simulink model "AFE_feed_VSI"  (Simulink 8.2)
settings: Solver=ode23tb  StartTime=0  StopTime=1  MaxStep=.5e-6  RelTol=1e-4  AbsTol=1e-5
values from neighbouring files (symbols this model uses):
  Ca = 41.308e-6    (= 4.1308e-05)    [VSI_AFE_parameters_stable.m]    (also in VSI_AFE_parameters_unstable.m)
  Cc = 41.308e-6    (= 4.1308e-05)    [VSI_AFE_parameters_stable.m]    (also in VSI_AFE_parameters_unstable.m)
  Cdc_afe = 35e-6    (= 3.5e-05)    [VSI_AFE_parameters_stable.m]    (also in VSI_AFE_parameters_unstable.m)
  Cdc_vsi = 10e-6    (= 1e-05)    [VSI_AFE_parameters_stable.m]    (also in VSI_AFE_parameters_unstable.m)
  DeadTime = 0.5e-6    (= 5e-07)    [VSI_AFE_parameters_stable.m]    (also in VSI_AFE_parameters_unstable.m)
  f = 400    [VSI_AFE_parameters_stable.m]    (also in VSI_AFE_parameters_unstable.m)
  FWPI_a1 = 26.7622    [VSI_AFE_parameters_stable.m]    (also in VSI_AFE_parameters_unstable.m)
  FWPI_a2 = -24.9784    [VSI_AFE_parameters_stable.m]    (also in VSI_AFE_parameters_unstable.m)
  Kii_AFE = 2.5598*270    (= 691.146)    [VSI_AFE_parameters_stable.m]    (also in VSI_AFE_parameters_unstable.m)
  Kii_VSI = 18.62*270    (= 5027.4)    [VSI_AFE_parameters_stable.m]    (also in VSI_AFE_parameters_unstable.m = 1507.95)
  Kiv_AFE = 6.9813    [VSI_AFE_parameters_stable.m]    (also in VSI_AFE_parameters_unstable.m = 3.49)
  Kiv_VSI = 125.6637    [VSI_AFE_parameters_stable.m]    (also in VSI_AFE_parameters_unstable.m = 41.89)
  Kpi_AFE = 0.0119*270    (= 3.213)    [VSI_AFE_parameters_stable.m]    (also in VSI_AFE_parameters_unstable.m)
  Kpi_VSI = 0.0102*270    (= 2.754)    [VSI_AFE_parameters_stable.m]    (also in VSI_AFE_parameters_unstable.m)
  Kpv_AFE = 0.022    [VSI_AFE_parameters_stable.m]    (also in VSI_AFE_parameters_unstable.m = 0.011)
  Kpv_VSI = 0.0779    [VSI_AFE_parameters_stable.m]    (also in VSI_AFE_parameters_unstable.m = 0.026)
  La = 962e-6    (= 0.000962)    [VSI_AFE_parameters_stable.m]    (also in VSI_AFE_parameters_unstable.m)
  Lb = 985e-6    (= 0.000985)    [VSI_AFE_parameters_stable.m]    (also in VSI_AFE_parameters_unstable.m)
  Lboost_a = 474e-6    (= 0.000474)    [VSI_AFE_parameters_stable.m]    (also in VSI_AFE_parameters_unstable.m)
  Lboost_b = 471e-6    (= 0.000471)    [VSI_AFE_parameters_stable.m]    (also in VSI_AFE_parameters_unstable.m)
  Lboost_c = 463e-6    (= 0.000463)    [VSI_AFE_parameters_stable.m]    (also in VSI_AFE_parameters_unstable.m)
  Lc = 972e-6    (= 0.000972)    [VSI_AFE_parameters_stable.m]    (also in VSI_AFE_parameters_unstable.m)
  LCa = 0.61e-6    (= 6.1e-07)    [VSI_AFE_parameters_stable.m]    (also in VSI_AFE_parameters_unstable.m)
  LCb = 0.61e-6    (= 6.1e-07)    [VSI_AFE_parameters_stable.m]    (also in VSI_AFE_parameters_unstable.m)
  LCc = 0.63e-6    (= 6.3e-07)    [VSI_AFE_parameters_stable.m]    (also in VSI_AFE_parameters_unstable.m)
  PWM_Cycle = 4000    [VSI_AFE_parameters_stable.m]    (also in VSI_AFE_parameters_unstable.m)
  R = 10    [VSI_AFE_parameters_stable.m]    (also in VSI_AFE_parameters_unstable.m)
  RCa = 0.051    [VSI_AFE_parameters_stable.m]    (also in VSI_AFE_parameters_unstable.m)
  RCb = 0.054    [VSI_AFE_parameters_stable.m]    (also in VSI_AFE_parameters_unstable.m)
  RCc = 0.052    [VSI_AFE_parameters_stable.m]    (also in VSI_AFE_parameters_unstable.m)
  RCdc_afe = 0.049    [VSI_AFE_parameters_stable.m]    (also in VSI_AFE_parameters_unstable.m)
  RCdc_vsi = 0.046    [VSI_AFE_parameters_stable.m]    (also in VSI_AFE_parameters_unstable.m)
  RLa = 0.123    [VSI_AFE_parameters_stable.m]    (also in VSI_AFE_parameters_unstable.m)
  RLb = 0.132    [VSI_AFE_parameters_stable.m]    (also in VSI_AFE_parameters_unstable.m)
  RLboost_a = 0.080    (= 0.08)    [VSI_AFE_parameters_stable.m]    (also in VSI_AFE_parameters_unstable.m)
  RLboost_c = 0.110    (= 0.11)    [VSI_AFE_parameters_stable.m]    (also in VSI_AFE_parameters_unstable.m)
  RLc = 0.089    [VSI_AFE_parameters_stable.m]    (also in VSI_AFE_parameters_unstable.m)
  Vfd = 0.75    [VSI_AFE_parameters_stable.m]    (also in VSI_AFE_parameters_unstable.m)
  Vfs = 1.0    (= 1)    [VSI_AFE_parameters_stable.m]    (also in VSI_AFE_parameters_unstable.m)
  Vsm = Vse*sqrt(2)    [VSI_AFE_parameters_stable.m]    (also in VSI_AFE_parameters_unstable.m)
undefined symbols (not defined in the file or in its folder): Cdc, Ldc
libraries: powerlib x42, cstblocks x10, simulink x4, powerlib_extras x1
settings Model: Creator=marko  LastModifiedBy=wenbo
settings SolverCC: MaxConsecutiveMinStep=10  ZeroCrossAlgorithm=Adaptive  AlgebraicLoopSolver=LineSearch
settings DataIOCC: LimitDataPoints=off  SaveOutput=off  SignalLogging=off  DSMLogging=off  SaveTime=off
settings DebuggingCC: IgnoredZcDiagnostic=none  FcnCallInpInsideContextMsg=EnableAllAsWarning

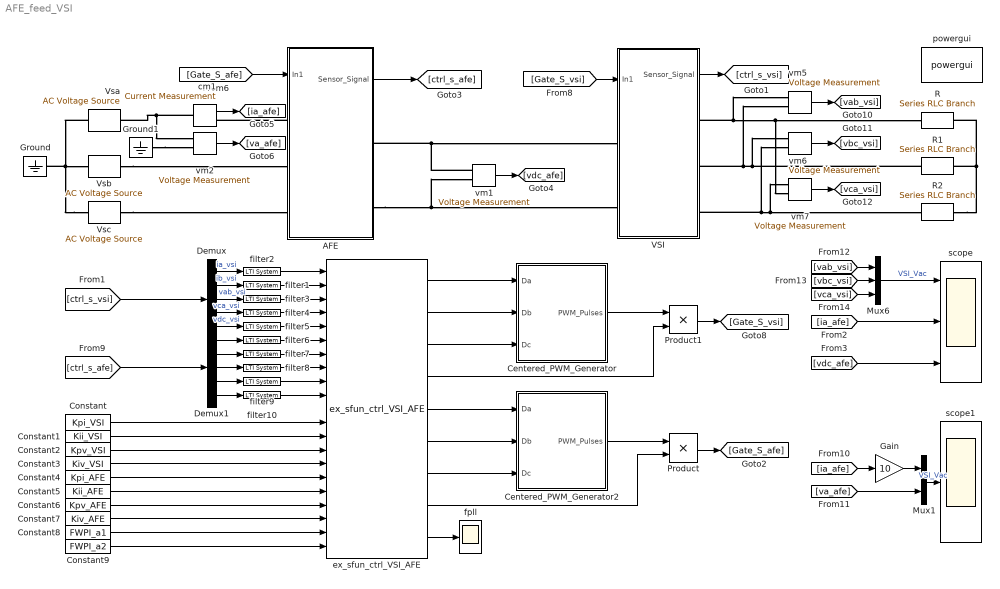
== system AFE_feed_VSI ==
  AFE : Subsystem
  Centered_PWM_Generator : Subsystem
  Centered_PWM_Generator2 : Subsystem
  Constant : Constant  Value=Kpi_VSI
  Constant1 : Constant  Value=Kii_VSI
  Constant2 : Constant  Value=Kpv_VSI
  Constant3 : Constant  Value=Kiv_VSI
  Constant4 : Constant  Value=Kpi_AFE
  Constant5 : Constant  Value=Kii_AFE
  Constant6 : Constant  Value=Kpv_AFE
  Constant7 : Constant  Value=Kiv_AFE
  Constant8 : Constant  Value=FWPI_a1
  Constant9 : Constant  Value=FWPI_a2
  Demux : Demux  Outputs=5
  Demux1 : Demux  Outputs=5
  Gain : Gain  Gain=10
  Ground : powerlib/Elements/Ground  LConnTagsString=a
  Ground1 : powerlib/Elements/Ground  LConnTagsString=a
  Mux1 : Mux  Inputs=2
  Mux6 : Mux  Inputs=3
  Product : Product  RndMeth=Zero
  Product1 : Product  RndMeth=Zero
  R : powerlib/Elements/Series RLC Branch  LConnTagsString=__new0  RConnTagsString=__new0  BranchType=R  Resistance=R  Inductance=Ldc  SetiL0=off  InitialCurrent=0  Capacitance=Cdc  Setx0=off  InitialVoltage=0  Measurements=None
  R1 : powerlib/Elements/Series RLC Branch  LConnTagsString=__new0  RConnTagsString=__new0  BranchType=R  Resistance=R  Inductance=Ldc  SetiL0=off  InitialCurrent=0  Capacitance=Cdc  Setx0=off  InitialVoltage=0  Measurements=None
  R2 : powerlib/Elements/Series RLC Branch  LConnTagsString=__new0  RConnTagsString=__new0  BranchType=R  Resistance=R  Inductance=Ldc  SetiL0=off  InitialCurrent=0  Capacitance=Cdc  Setx0=off  InitialVoltage=0  Measurements=None
  VSI : Subsystem
  Vsa : powerlib/Electrical Sources/AC Voltage Source  Amplitude=Vsm  Phase=90  Frequency=f  SampleTime=0  Measurements=None
  Vsb : powerlib/Electrical Sources/AC Voltage Source  Amplitude=Vsm  Phase=90-120  Frequency=f  SampleTime=0  Measurements=None
  Vsc : powerlib/Electrical Sources/AC Voltage Source  Amplitude=Vsm  Phase=90+120  Frequency=f  SampleTime=0  Measurements=None
  cm1 : powerlib/Measurements/Current Measurement  PhasorSimulation=off  OutputType=Complex  PSBequivalent=0
  ex_sfun_ctrl_VSI_AFE : S-Function  FunctionName=ex_sfun_ctrl_VSI_AFE  EnableBusSupport=off
  filter{1..3,6..8} (6 alike) : cstblocks/LTI System  sys=tf_i_filter  IC=[]
  filter{4..5,9..10} (4 alike) : cstblocks/LTI System  sys=tf_v_filter  IC=[]
  fpll : Scope
      settings: YMin=-500  YMax=50  SaveName=ia_L1
  powergui : powerlib/powergui  Priority=1  SimulationMode=Continuous  SolverType=Tustin  SampleTime=50e-6  frequency=60  SPID=on  DisableSnubberDevices=off  DisableRonSwitches=off  DisableVfSwitches=off  SwTol=0  Interpol=off  DisplayEquations=off  frequencyindice=0  Pbase=100e6  ErrMax=1e-4  Iterations=50  UnitsV=kV  UnitsW=MW  FunctionMessages=off  echomessages=off  HookPort=off  EnableUseOfTLC=off  x0status=blocks  RestoreLinks=warning  ResistiveCurrentMeasurement=off  Frange=[0:2:500]  Ylog=off  Xlog=on  ShowGrid=off  save=off  variable=ZData  structure=ia_L  ZoomFFT=on  StartTime=0.1  cycles=1  DisplayStyle=1  fundamental=400  FreqAxis=off  MaxFrequency=100000  frequencyindicesteady=400  RmsSteady=1  display=off  Ts=0  methode=off
  scope : Scope  NumInputPorts=3
      settings: YMin=-200~-15~0  YMax=200~30~450  SaveName=va_ia  MaxDataPoints=2000000
  scope1 : Scope
      settings: YMin=-800  YMax=900  SaveName=va_ia1  MaxDataPoints=2000000
  vm{1..2,5..7} (5 alike) : powerlib/Measurements/Voltage Measurement  PhasorSimulation=off  OutputType=Complex  PSBequivalent=0
  wires:
  vm5/1 -> [vab_vsi]
  vm6/1 -> [vbc_vsi]
  vm7/1 -> [vca_vsi]
  [vab_vsi] -> Mux6/1
  [vbc_vsi] -> Mux6/2
  [vca_vsi] -> Mux6/3
  Mux6/1 -> scope/1  "VSI_Vac"
  VSI/1(Sensor_Signal) -> [ctrl_s_vsi]
  [Gate_S_vsi] -> VSI/1(In1)
  [ctrl_s_afe] -> Demux1/1
  [Gate_S_afe] -> AFE/1(In1)
  AFE/1(Sensor_Signal) -> [ctrl_s_afe]
  ex_sfun_ctrl_VSI_AFE/1 -> Centered_PWM_Generator/1(Da)
  ex_sfun_ctrl_VSI_AFE/2 -> Centered_PWM_Generator/2(Db)
  ex_sfun_ctrl_VSI_AFE/3 -> Centered_PWM_Generator/3(Dc)
  Centered_PWM_Generator2/1(PWM_Pulses) -> Product/1
  Product/1 -> [Gate_S_afe]
  vm1/1 -> [vdc_afe]
  cm1/1 -> [ia_afe]
  [ia_afe] -> scope/2
  [vdc_afe] -> scope/3
  [ctrl_s_vsi] -> Demux/1
  Demux/1 -> filter2/1  "ia_vsi"
  Demux/2 -> filter1/1  "ib_vsi"
  Demux/3 -> filter3/1  "vab_vsi"
  Demux/4 -> filter4/1  "vca_vsi"
  Demux/5 -> filter5/1  "vdc_vsi"
  Demux1/1 -> filter6/1
  Demux1/2 -> filter7/1
  Demux1/3 -> filter8/1
  Demux1/4 -> filter9/1
  Demux1/5 -> filter10/1
  Constant/1 -> ex_sfun_ctrl_VSI_AFE/12
  Constant1/1 -> ex_sfun_ctrl_VSI_AFE/13
  Constant2/1 -> ex_sfun_ctrl_VSI_AFE/14
  Constant3/1 -> ex_sfun_ctrl_VSI_AFE/15
  Constant4/1 -> ex_sfun_ctrl_VSI_AFE/16
  Constant5/1 -> ex_sfun_ctrl_VSI_AFE/17
  Constant6/1 -> ex_sfun_ctrl_VSI_AFE/18
  Constant7/1 -> ex_sfun_ctrl_VSI_AFE/19
  Constant8/1 -> ex_sfun_ctrl_VSI_AFE/20
  Constant9/1 -> ex_sfun_ctrl_VSI_AFE/21
  filter2/1 -> ex_sfun_ctrl_VSI_AFE/1
  filter1/1 -> ex_sfun_ctrl_VSI_AFE/2
  filter3/1 -> ex_sfun_ctrl_VSI_AFE/3
  filter4/1 -> ex_sfun_ctrl_VSI_AFE/4
  filter5/1 -> ex_sfun_ctrl_VSI_AFE/5
  filter6/1 -> ex_sfun_ctrl_VSI_AFE/6
  filter7/1 -> ex_sfun_ctrl_VSI_AFE/7
  filter8/1 -> ex_sfun_ctrl_VSI_AFE/8
  filter9/1 -> ex_sfun_ctrl_VSI_AFE/9
  filter10/1 -> ex_sfun_ctrl_VSI_AFE/10
  vm2/1 -> [va_afe]
  ex_sfun_ctrl_VSI_AFE/9 -> fpll/1
  ex_sfun_ctrl_VSI_AFE/5 -> Centered_PWM_Generator2/1(Da)
  ex_sfun_ctrl_VSI_AFE/6 -> Centered_PWM_Generator2/2(Db)
  ex_sfun_ctrl_VSI_AFE/7 -> Centered_PWM_Generator2/3(Dc)
  ex_sfun_ctrl_VSI_AFE/8 -> Product/2
  Product1/1 -> [Gate_S_vsi]
  Centered_PWM_Generator/1(PWM_Pulses) -> Product1/1
  ex_sfun_ctrl_VSI_AFE/4 -> Product1/2
  Mux1/1 -> scope1/1  "VSI_Vac"
  [ia_afe] -> Gain/1
  [va_afe] -> Mux1/2
  Gain/1 -> Mux1/1
  connections:
  VSI/RConn1 -- vm5/LConn1 -- R/RConn1 -- vm7/LConn2
  R1/RConn1 -- VSI/RConn2 -- vm5/LConn2 -- vm6/LConn1
  VSI/RConn3 -- vm6/LConn2 -- R2/RConn1 -- vm7/LConn1
  AFE/RConn2 -- VSI/LConn2 -- vm1/LConn2
  Vsc/LConn1 -- Vsb/LConn1 -- Vsa/LConn1 -- Ground/LConn1
  Vsb/RConn1 -- AFE/LConn2
  Vsc/RConn1 -- AFE/LConn3
  AFE/LConn1 -- cm1/RConn1
  cm1/LConn1 -- Vsa/RConn1 -- vm2/LConn1
  Ground1/LConn1 -- vm2/LConn2
  R2/LConn1 -- R/LConn1 -- R1/LConn1
  vm1/LConn1 -- VSI/LConn1 -- AFE/RConn1

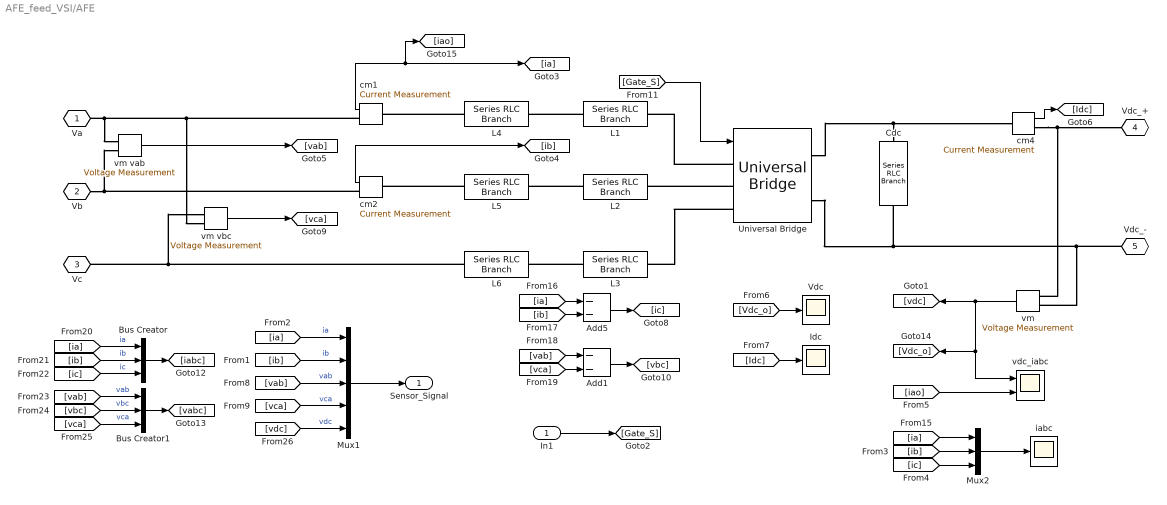
== system AFE_feed_VSI/AFE ==
  In1 : Inport
  Add1 : Sum  Inputs=--
  Add5 : Sum  Inputs=--
  Bus Creator : BusCreator  Inputs=3
  Bus Creator1 : BusCreator  Inputs=3
  Cdc : powerlib/Elements/Series RLC Branch  LConnTagsString=__new0  RConnTagsString=__new0  BranchType=RC  Resistance=RCdc_afe  Inductance=Ldc  SetiL0=off  InitialCurrent=0  Capacitance=Cdc_afe  Setx0=off  InitialVoltage=0  Measurements=None
  Idc : Scope
      settings: YMin=1.813  YMax=1.8195  SaveName=vdc_matlab1
  L1 : powerlib/Elements/Series RLC Branch  LConnTagsString=__new0  RConnTagsString=__new0  BranchType=L  Resistance=RLa  Inductance=Lboost_a  SetiL0=off  InitialCurrent=0  Capacitance=1e-6  Setx0=off  InitialVoltage=0  Measurements=None
  L2 : powerlib/Elements/Series RLC Branch  LConnTagsString=__new0  RConnTagsString=__new0  BranchType=L  Resistance=RLa  Inductance=Lboost_b  SetiL0=off  InitialCurrent=0  Capacitance=1e-6  Setx0=off  InitialVoltage=0  Measurements=None
  L3 : powerlib/Elements/Series RLC Branch  LConnTagsString=__new0  RConnTagsString=__new0  BranchType=L  Resistance=RLa  Inductance=Lboost_c  SetiL0=off  InitialCurrent=0  Capacitance=1e-6  Setx0=off  InitialVoltage=0  Measurements=None
  L4 : powerlib/Elements/Series RLC Branch  LConnTagsString=__new0  RConnTagsString=__new0  BranchType=R  Resistance=RLboost_a  Inductance=La  SetiL0=off  InitialCurrent=0  Capacitance=1e-6  Setx0=off  InitialVoltage=0  Measurements=None
  L5 : powerlib/Elements/Series RLC Branch  LConnTagsString=__new0  RConnTagsString=__new0  BranchType=R  Resistance=Lboost_b  Inductance=La  SetiL0=off  InitialCurrent=0  Capacitance=1e-6  Setx0=off  InitialVoltage=0  Measurements=None
  L6 : powerlib/Elements/Series RLC Branch  LConnTagsString=__new0  RConnTagsString=__new0  BranchType=R  Resistance=RLboost_c  Inductance=La  SetiL0=off  InitialCurrent=0  Capacitance=1e-6  Setx0=off  InitialVoltage=0  Measurements=None
  Mux1 : Mux  Inputs=5
  Mux2 : Mux  Inputs=3
  Universal Bridge : powerlib/Power Electronics/Universal Bridge  Arms=3  SnubberResistance=inf  SnubberCapacitance=inf  Device=IGBT / Diodes  Ron=Rsd  Lon=0  ForwardVoltages=[Vfs Vfd]  ForwardVoltage=0  GTOparameters=[ 10e-6 , 20e-6 ]  IGBTparameters=[ 0, 0 ]  Measurements=None  Measurements_2=None  converterType=Rectifier
  Vdc : Scope
      settings: TimeRange=0.3  YMin=0  YMax=300  SaveName=vdc_matlab
  cm1 : powerlib/Measurements/Current Measurement  PhasorSimulation=off  OutputType=Complex  PSBequivalent=0
  cm2 : powerlib/Measurements/Current Measurement  PhasorSimulation=off  OutputType=Complex  PSBequivalent=0
  cm4 : powerlib/Measurements/Current Measurement  PhasorSimulation=off  OutputType=Complex  PSBequivalent=0
  iabc : Scope
      settings: TimeRange=0.06  YMin=-8  YMax=8  SaveName=iabc_L
  vdc_iabc : Scope  NumInputPorts=2
      settings: TimeRange=0.3  YMin=131~-2  YMax=137~2  SaveName=iabc_L1
  vm : powerlib/Measurements/Voltage Measurement  PhasorSimulation=off  OutputType=Complex  PSBequivalent=0
  vm vab : powerlib/Measurements/Voltage Measurement  PhasorSimulation=off  OutputType=Complex  PSBequivalent=0
  vm vbc : powerlib/Measurements/Voltage Measurement  PhasorSimulation=off  OutputType=Complex  PSBequivalent=0
  Va : PMIOPort  Tag=PMCPort  Port=1  Side=Left
  Vb : PMIOPort  Tag=PMCPort  Port=2  Side=Left
  Vc : PMIOPort  Tag=PMCPort  Port=3  Side=Left
  Vdc_+ : PMIOPort  Tag=PMCPort  Port=4  Side=Right
  Vdc_- : PMIOPort  Tag=PMCPort  Port=5  Side=Right
  Sensor_Signal : Outport
  wires:
  [Vdc_o] -> Vdc/1
  [Idc] -> Idc/1
  [Gate_S] -> Universal Bridge/1
  [ia] -> Bus Creator/1  "ia"
  [ib] -> Bus Creator/2  "ib"
  [ic] -> Bus Creator/3  "ic"
  Bus Creator/1 -> [iabc]
  [vab] -> Bus Creator1/1  "vab"
  [vbc] -> Bus Creator1/2  "vbc"
  [vca] -> Bus Creator1/3  "vca"
  Bus Creator1/1 -> [vabc]
  cm4/1 -> [Idc]
  Mux2/1 -> iabc/1
  [ia] -> Mux2/1
  [ib] -> Mux2/2
  [ic] -> Mux2/3
  cm1/1 -> [iao], [ia]
  cm2/1 -> [ib]
  vm vab/1 -> [vab]
  vm vbc/1 -> [vca]
  [iao] -> vdc_iabc/2
  vm/1 -> [Vdc_o], vdc_iabc/1, [vdc]
  [ia] -> Mux1/1  "ia"
  [ib] -> Mux1/2  "ib"
  [vab] -> Mux1/3  "vab"
  [vca] -> Mux1/4  "vca"
  [vdc] -> Mux1/5  "vdc"
  Mux1/1 -> Sensor_Signal/1
  In1/1 -> [Gate_S]
  Add5/1 -> [ic]
  [ia] -> Add5/1
  [ib] -> Add5/2
  Add1/1 -> [vbc]
  [vab] -> Add1/1
  [vca] -> Add1/2
  connections:
  Universal Bridge/LConn1 -- L1/RConn1
  Universal Bridge/LConn2 -- L2/RConn1
  Universal Bridge/LConn3 -- L3/RConn1
  vm vab/LConn1 -- cm1/RConn1 -- vm vbc/LConn2 -- Va/RConn1
  cm2/RConn1 -- Vb/RConn1 -- vm vab/LConn2
  L6/LConn1 -- Vc/RConn1 -- vm vbc/LConn1
  cm4/RConn1 -- Vdc_+/RConn1 -- vm/LConn1
  Vdc_-/RConn1 -- Universal Bridge/RConn2 -- Cdc/RConn1 -- vm/LConn2
  L1/LConn1 -- L4/RConn1
  L4/LConn1 -- cm1/LConn1
  L2/LConn1 -- L5/RConn1
  L5/LConn1 -- cm2/LConn1
  L3/LConn1 -- L6/RConn1
  Universal Bridge/RConn1 -- cm4/LConn1 -- Cdc/LConn1

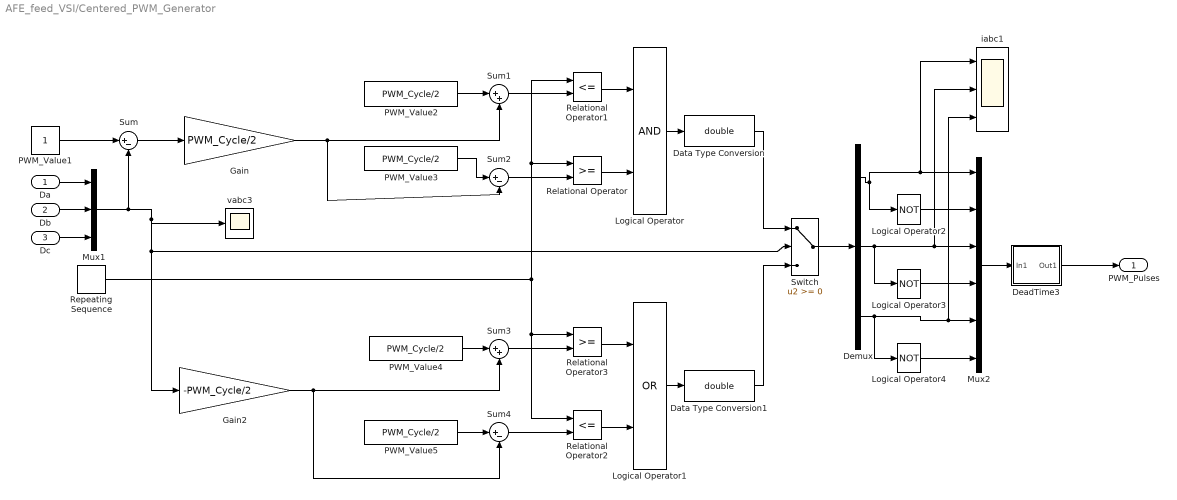
== system AFE_feed_VSI/Centered_PWM_Generator ==
  Da : Inport
  Db : Inport  Port=2
  Dc : Inport  Port=3
  Data Type Conversion : DataTypeConversion  OutDataTypeStr=double
  Data Type Conversion1 : DataTypeConversion  OutDataTypeStr=double
  DeadTime3 : Subsystem
  Demux : Demux  Outputs=3
  Gain : Gain  Gain=PWM_Cycle/2
  Gain2 : Gain  Gain=-PWM_Cycle/2
  Logical Operator : Logic  AllPortsSameDT=off  OutDataTypeStr=boolean
  Logical Operator1 : Logic  Operator=OR  AllPortsSameDT=off  OutDataTypeStr=boolean
  Logical Operator2 : Logic  Operator=NOT  OutDataTypeStr=float('double')
  Logical Operator3 : Logic  Operator=NOT  OutDataTypeStr=float('double')
  Logical Operator4 : Logic  Operator=NOT  OutDataTypeStr=float('double')
  Mux1 : Mux  Inputs=3
  Mux2 : Mux  Inputs=6
  PWM_Value1 : Constant
  PWM_Value{2..5} (4 alike) : Constant  Value=PWM_Cycle/2
  Relational Operator : RelationalOperator  OutDataTypeStr=boolean
  Relational Operator1 : RelationalOperator  Operator=<=  OutDataTypeStr=boolean
  Relational Operator2 : RelationalOperator  Operator=<=  OutDataTypeStr=boolean
  Relational Operator3 : RelationalOperator  OutDataTypeStr=boolean
  Repeating Sequence : simulink/Sources/Repeating Sequence  rep_seq_t="[0  (PWM_Cycle*12.5e-9)]"  rep_seq_y=[0 PWM_Cycle]
  Sum : Sum  Inputs=|+-
  Sum1 : Sum  Inputs=|++
  Sum2 : Sum  Inputs=|+-
  Sum3 : Sum  Inputs=|++
  Sum4 : Sum  Inputs=|+-
  Switch : Switch
  iabc1 : Scope  NumInputPorts=3
      settings: TimeRange=0.02  YMin=-9~-5~-5  YMax=8~5~5  SaveName=iabc_L2
  vabc3 : Scope
      settings: TimeRange=0.01  YMin=0.275  YMax=0.725  SaveName=vabcll1
  PWM_Pulses : Outport
  wires:
  Logical Operator4/1 -> Mux2/6
  Demux/3 -> Logical Operator4/1, Mux2/5, iabc1/3
  Logical Operator3/1 -> Mux2/4
  Demux/2 -> Logical Operator3/1, Mux2/3, iabc1/2
  Logical Operator2/1 -> Mux2/2
  Demux/1 -> Logical Operator2/1, Mux2/1, iabc1/1
  Mux2/1 -> DeadTime3/1(In1)
  Dc/1 -> Mux1/3
  Db/1 -> Mux1/2
  Da/1 -> Mux1/1
  Mux1/1 -> Sum/2, Switch/2, Gain2/1, vabc3/1
  Switch/1 -> Demux/1
  Data Type Conversion1/1 -> Switch/3
  Gain2/1 -> Sum3/2, Sum4/2
  Logical Operator1/1 -> Data Type Conversion1/1
  Relational Operator2/1 -> Logical Operator1/2
  Relational Operator3/1 -> Logical Operator1/1
  Sum3/1 -> Relational Operator3/2
  Sum4/1 -> Relational Operator2/2
  PWM_Value5/1 -> Sum4/1
  PWM_Value4/1 -> Sum3/1
  Data Type Conversion/1 -> Switch/1
  Logical Operator/1 -> Data Type Conversion/1
  Relational Operator/1 -> Logical Operator/2
  Relational Operator1/1 -> Logical Operator/1
  Sum1/1 -> Relational Operator1/2
  Sum2/1 -> Relational Operator/2
  PWM_Value3/1 -> Sum2/1
  Gain/1 -> Sum2/2, Sum1/2
  Sum/1 -> Gain/1
  PWM_Value1/1 -> Sum/1
  Repeating Sequence/1 -> Relational Operator1/1, Relational Operator/1, Relational Operator3/1, Relational Operator2/1
  DeadTime3/1(Out1) -> PWM_Pulses/1
  PWM_Value2/1 -> Sum1/1

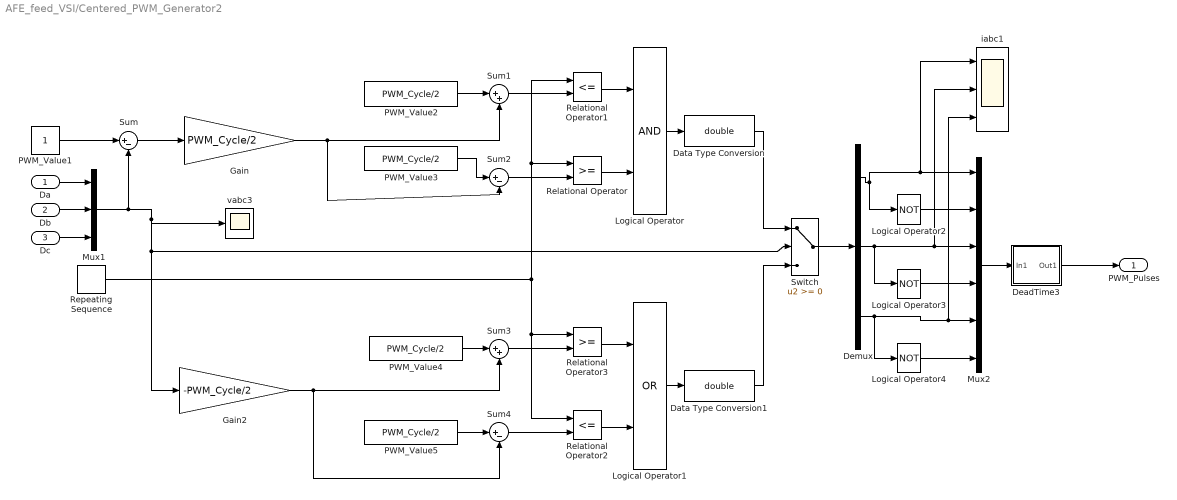
== system AFE_feed_VSI/Centered_PWM_Generator2 ==
  Da : Inport
  Db : Inport  Port=2
  Dc : Inport  Port=3
  Data Type Conversion : DataTypeConversion  OutDataTypeStr=double
  Data Type Conversion1 : DataTypeConversion  OutDataTypeStr=double
  DeadTime3 : Subsystem
  Demux : Demux  Outputs=3
  Gain : Gain  Gain=PWM_Cycle/2
  Gain2 : Gain  Gain=-PWM_Cycle/2
  Logical Operator : Logic  AllPortsSameDT=off  OutDataTypeStr=boolean
  Logical Operator1 : Logic  Operator=OR  AllPortsSameDT=off  OutDataTypeStr=boolean
  Logical Operator2 : Logic  Operator=NOT  OutDataTypeStr=float('double')
  Logical Operator3 : Logic  Operator=NOT  OutDataTypeStr=float('double')
  Logical Operator4 : Logic  Operator=NOT  OutDataTypeStr=float('double')
  Mux1 : Mux  Inputs=3
  Mux2 : Mux  Inputs=6
  PWM_Value1 : Constant
  PWM_Value{2..5} (4 alike) : Constant  Value=PWM_Cycle/2
  Relational Operator : RelationalOperator  OutDataTypeStr=boolean
  Relational Operator1 : RelationalOperator  Operator=<=  OutDataTypeStr=boolean
  Relational Operator2 : RelationalOperator  Operator=<=  OutDataTypeStr=boolean
  Relational Operator3 : RelationalOperator  OutDataTypeStr=boolean
  Repeating Sequence : simulink/Sources/Repeating Sequence  rep_seq_t="[0  (PWM_Cycle*12.5e-9)]"  rep_seq_y=[0 PWM_Cycle]
  Sum : Sum  Inputs=|+-
  Sum1 : Sum  Inputs=|++
  Sum2 : Sum  Inputs=|+-
  Sum3 : Sum  Inputs=|++
  Sum4 : Sum  Inputs=|+-
  Switch : Switch
  iabc1 : Scope  NumInputPorts=3
      settings: TimeRange=0.02  YMin=-9~-5~-5  YMax=8~5~5  SaveName=iabc_L2
  vabc3 : Scope
      settings: TimeRange=0.01  YMin=-35  YMax=35  SaveName=vabcll1
  PWM_Pulses : Outport
  wires:
  Logical Operator4/1 -> Mux2/6
  Demux/3 -> Logical Operator4/1, Mux2/5, iabc1/3
  Logical Operator3/1 -> Mux2/4
  Demux/2 -> Logical Operator3/1, Mux2/3, iabc1/2
  Logical Operator2/1 -> Mux2/2
  Demux/1 -> Logical Operator2/1, Mux2/1, iabc1/1
  Mux2/1 -> DeadTime3/1(In1)
  Dc/1 -> Mux1/3
  Db/1 -> Mux1/2
  Da/1 -> Mux1/1
  Mux1/1 -> Sum/2, Switch/2, Gain2/1, vabc3/1
  Switch/1 -> Demux/1
  Data Type Conversion1/1 -> Switch/3
  Gain2/1 -> Sum3/2, Sum4/2
  Logical Operator1/1 -> Data Type Conversion1/1
  Relational Operator2/1 -> Logical Operator1/2
  Relational Operator3/1 -> Logical Operator1/1
  Sum3/1 -> Relational Operator3/2
  Sum4/1 -> Relational Operator2/2
  PWM_Value5/1 -> Sum4/1
  PWM_Value4/1 -> Sum3/1
  Data Type Conversion/1 -> Switch/1
  Logical Operator/1 -> Data Type Conversion/1
  Relational Operator/1 -> Logical Operator/2
  Relational Operator1/1 -> Logical Operator/1
  Sum1/1 -> Relational Operator1/2
  Sum2/1 -> Relational Operator/2
  PWM_Value3/1 -> Sum2/1
  Gain/1 -> Sum2/2, Sum1/2
  Sum/1 -> Gain/1
  PWM_Value1/1 -> Sum/1
  Repeating Sequence/1 -> Relational Operator1/1, Relational Operator/1, Relational Operator3/1, Relational Operator2/1
  DeadTime3/1(Out1) -> PWM_Pulses/1
  PWM_Value2/1 -> Sum1/1

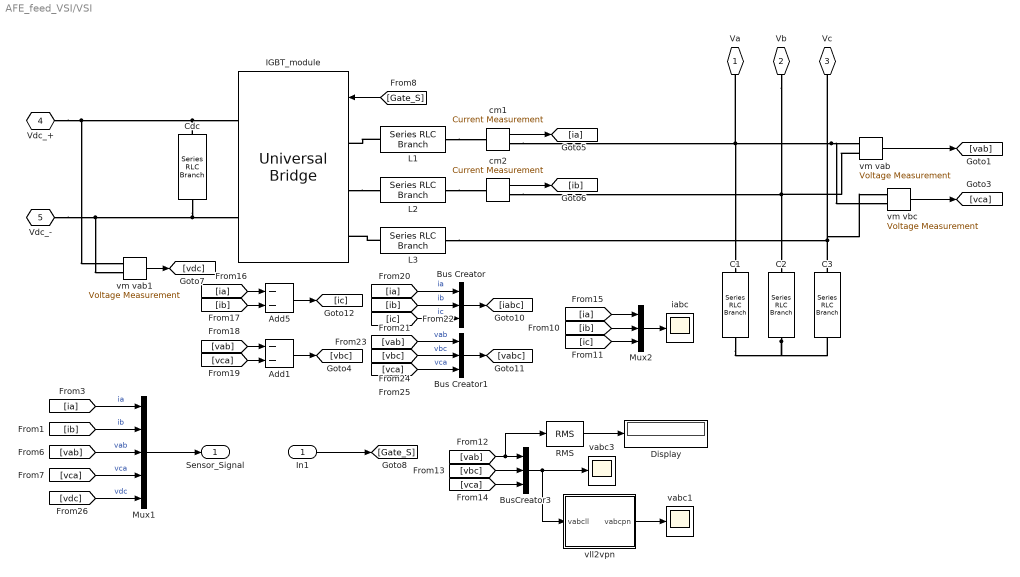
== system AFE_feed_VSI/VSI ==
  In1 : Inport
  Add1 : Sum  Inputs=--
  Add5 : Sum  Inputs=--
  Bus Creator : BusCreator  Inputs=3
  Bus Creator1 : BusCreator  Inputs=3
  BusCreator3 : BusCreator  Inputs=3
  C1 : powerlib/Elements/Series RLC Branch  LConnTagsString=__new0  RConnTagsString=__new0  BranchType=RC  Resistance=RCa  Inductance=LCa  SetiL0=off  InitialCurrent=0  Capacitance=Ca  Setx0=off  InitialVoltage=0  Measurements=None
  C2 : powerlib/Elements/Series RLC Branch  LConnTagsString=__new0  RConnTagsString=__new0  BranchType=RC  Resistance=RCb  Inductance=LCb  SetiL0=off  InitialCurrent=0  Capacitance=Cc  Setx0=off  InitialVoltage=0  Measurements=None
  C3 : powerlib/Elements/Series RLC Branch  LConnTagsString=__new0  RConnTagsString=__new0  BranchType=RC  Resistance=RCc  Inductance=LCc  SetiL0=off  InitialCurrent=0  Capacitance=Cc  Setx0=off  InitialVoltage=0  Measurements=None
  Cdc : powerlib/Elements/Series RLC Branch  LConnTagsString=__new0  RConnTagsString=__new0  BranchType=RC  Resistance=RCdc_vsi  Inductance=Ldc  SetiL0=off  InitialCurrent=0  Capacitance=Cdc_vsi  Setx0=off  InitialVoltage=0  Measurements=None
  Display : Display
  IGBT_module : powerlib/Power Electronics/Universal Bridge  Arms=3  SnubberResistance=inf  SnubberCapacitance=inf  Device=IGBT / Diodes  Ron=Rsd  Lon=0  ForwardVoltages=[Vfs Vfd]  ForwardVoltage=0  GTOparameters=[ 10e-6 , 20e-6 ]  IGBTparameters=[ 0, 0 ]  Measurements=None  Measurements_2=None  converterType=Rectifier
  L1 : powerlib/Elements/Series RLC Branch  LConnTagsString=__new0  RConnTagsString=__new0  BranchType=RL  Resistance=RLa  Inductance=La  SetiL0=off  InitialCurrent=0  Capacitance=1e-6  Setx0=off  InitialVoltage=0  Measurements=None
  L2 : powerlib/Elements/Series RLC Branch  LConnTagsString=__new0  RConnTagsString=__new0  BranchType=RL  Resistance=RLb  Inductance=Lb  SetiL0=off  InitialCurrent=0  Capacitance=1e-6  Setx0=off  InitialVoltage=0  Measurements=None
  L3 : powerlib/Elements/Series RLC Branch  LConnTagsString=__new0  RConnTagsString=__new0  BranchType=RL  Resistance=RLc  Inductance=Lc  SetiL0=off  InitialCurrent=0  Capacitance=1e-6  Setx0=off  InitialVoltage=0  Measurements=None
  Mux1 : Mux  Inputs=5
  Mux2 : Mux  Inputs=3
  RMS : powerlib_extras/Measurements/RMS  f1=400
  cm1 : powerlib/Measurements/Current Measurement  PhasorSimulation=off  OutputType=Complex  PSBequivalent=0
  cm2 : powerlib/Measurements/Current Measurement  PhasorSimulation=off  OutputType=Complex  PSBequivalent=0
  iabc : Scope
      settings: TimeRange=0.06  YMin=-10  YMax=10  SaveName=iabc_L
  vabc1 : Scope
      settings: TimeRange=0.01  YMin=-80  YMax=80  SaveName=vabc
  vabc3 : Scope
      settings: TimeRange=0.06  YMin=-300  YMax=225  SaveName=vabcll
  vll2vpn : Subsystem
  vm vab : powerlib/Measurements/Voltage Measurement  PhasorSimulation=off  OutputType=Complex  PSBequivalent=0
  vm vab1 : powerlib/Measurements/Voltage Measurement  PhasorSimulation=off  OutputType=Complex  PSBequivalent=0
  vm vbc : powerlib/Measurements/Voltage Measurement  PhasorSimulation=off  OutputType=Complex  PSBequivalent=0
  Va : PMIOPort  Tag=PMCPort  Port=1  Side=Right
  Vb : PMIOPort  Tag=PMCPort  Port=2  Side=Right
  Vc : PMIOPort  Tag=PMCPort  Port=3  Side=Right
  Vdc_+ : PMIOPort  Tag=PMCPort  Port=4  Side=Left
  Vdc_- : PMIOPort  Tag=PMCPort  Port=5  Side=Left
  Sensor_Signal : Outport
  wires:
  cm1/1 -> [ia]
  [Gate_S] -> IGBT_module/1
  Mux2/1 -> iabc/1
  BusCreator3/1 -> vabc3/1, vll2vpn/1(vabcll)
  [ia] -> Mux2/1
  [ib] -> Mux2/2
  [ic] -> Mux2/3
  [vab] -> BusCreator3/1, RMS/1
  [vbc] -> BusCreator3/2
  [vca] -> BusCreator3/3
  [ia] -> Bus Creator/1  "ia"
  [ib] -> Bus Creator/2  "ib"
  [ic] -> Bus Creator/3  "ic"
  Bus Creator/1 -> [iabc]
  [vab] -> Bus Creator1/1  "vab"
  [vbc] -> Bus Creator1/2  "vbc"
  [vca] -> Bus Creator1/3  "vca"
  Bus Creator1/1 -> [vabc]
  vll2vpn/1(vabcpn) -> vabc1/1
  RMS/1 -> Display/1
  cm2/1 -> [ib]
  vm vab/1 -> [vab]
  vm vbc/1 -> [vca]
  vm vab1/1 -> [vdc]
  [ia] -> Mux1/1  "ia"
  [ib] -> Mux1/2  "ib"
  [vab] -> Mux1/3  "vab"
  [vca] -> Mux1/4  "vca"
  [vdc] -> Mux1/5  "vdc"
  Mux1/1 -> Sensor_Signal/1
  In1/1 -> [Gate_S]
  Add5/1 -> [ic]
  [ia] -> Add5/1
  [ib] -> Add5/2
  Add1/1 -> [vbc]
  [vab] -> Add1/1
  [vca] -> Add1/2
  connections:
  Va/RConn1 -- C1/LConn1 -- cm1/RConn1 -- vm vab/LConn1 -- vm vbc/LConn2
  C3/RConn1 -- C1/RConn1 -- C2/RConn1
  vm vab/LConn2 -- Vb/RConn1 -- cm2/RConn1 -- C2/LConn1
  L1/LConn1 -- IGBT_module/LConn1
  L1/RConn1 -- cm1/LConn1
  L2/RConn1 -- cm2/LConn1
  IGBT_module/LConn2 -- L2/LConn1
  L3/LConn1 -- IGBT_module/LConn3
  Vdc_+/RConn1 -- Cdc/LConn1 -- IGBT_module/RConn1 -- vm vab1/LConn1
  Vdc_-/RConn1 -- Cdc/RConn1 -- IGBT_module/RConn2 -- vm vab1/LConn2
  Vc/RConn1 -- vm vbc/LConn1 -- L3/RConn1 -- C3/LConn1

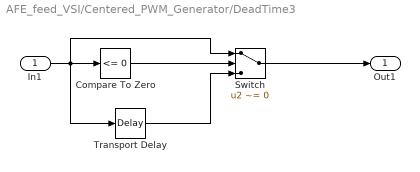
== system AFE_feed_VSI/Centered_PWM_Generator/DeadTime3 ==
  In1 : Inport
  Compare To Zero : simulink/Logic and Bit Operations/Compare To Zero  relop=<=  OutDataTypeStr=uint8
  Switch : Switch  Criteria=u2 ~= 0
  Transport Delay : TransportDelay  DelayTime=DeadTime  BufferSize=2048*16  FixedBuffer=on
  Out1 : Outport
  wires:
  Switch/1 -> Out1/1
  Compare To Zero/1 -> Switch/2
  Transport Delay/1 -> Switch/3
  In1/1 -> Transport Delay/1, Compare To Zero/1, Switch/1

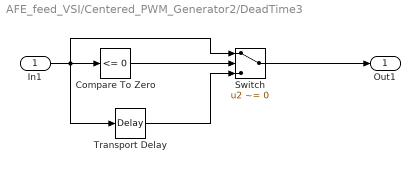
== system AFE_feed_VSI/Centered_PWM_Generator2/DeadTime3 ==
  In1 : Inport
  Compare To Zero : simulink/Logic and Bit Operations/Compare To Zero  relop=<=  OutDataTypeStr=uint8
  Switch : Switch  Criteria=u2 ~= 0
  Transport Delay : TransportDelay  DelayTime=DeadTime  BufferSize=2048*16  FixedBuffer=on
  Out1 : Outport
  wires:
  Switch/1 -> Out1/1
  Compare To Zero/1 -> Switch/2
  Transport Delay/1 -> Switch/3
  In1/1 -> Transport Delay/1, Compare To Zero/1, Switch/1

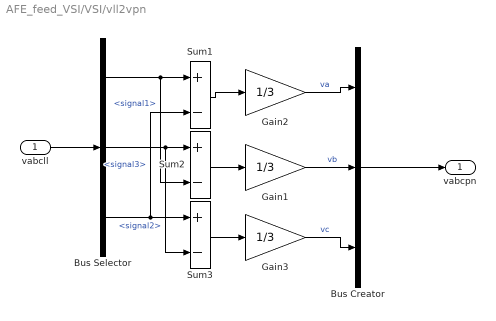
== system AFE_feed_VSI/VSI/vll2vpn ==
  vabcll : Inport
  Bus Creator : BusCreator  Inputs=3
  Bus Selector : BusSelector
  Gain1 : Gain  Gain=1/3
  Gain2 : Gain  Gain=1/3
  Gain3 : Gain  Gain=1/3
  Sum1 : Sum  Inputs=+-
  Sum2 : Sum  Inputs=+-
  Sum3 : Sum  Inputs=+-
  vabcpn : Outport
  wires:
  Bus Creator/1 -> vabcpn/1
  vabcll/1 -> Bus Selector/1
  Bus Selector/1 -> Sum1/1, Sum2/2  "<signal1>"
  Bus Selector/3 -> Sum1/2, Sum3/1  "<signal3>"
  Sum1/1 -> Gain2/1
  Bus Selector/2 -> Sum2/1, Sum3/2  "<signal2>"
  Sum2/1 -> Gain1/1
  Sum3/1 -> Gain3/1
  Gain2/1 -> Bus Creator/1  "va"
  Gain1/1 -> Bus Creator/2  "vb"
  Gain3/1 -> Bus Creator/3  "vc"
